simulink model "BLTSIM_MASTER_MODEL"  (R2021b)
settings: Solver=VariableStepAuto  StartTime=0.0  StopTime=Simulation.StopTime  RelTol=1e-3
undefined symbols (not defined in the file or in its folder): initialStateVector, vehicle
libraries: telemetrySubsystem x2, equationsOfMotionSubsystem x1, ForcesSubsystem x1, groundCheckSubsystem x1, outputHandlingSubsytem x1
settings Model: SnapshotInterval=1  Creator=mat  LastModifiedBy=mat

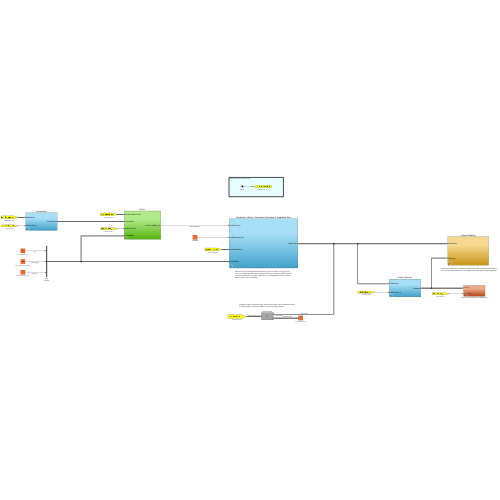
[thumbnail: Simulink's stored preview of the top-level diagram]
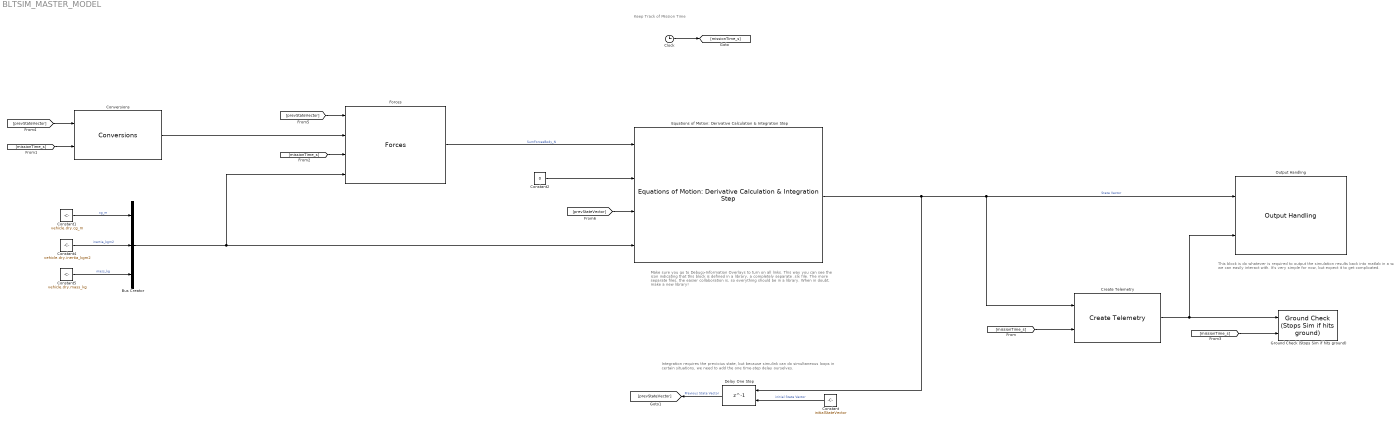
== system BLTSIM_MASTER_MODEL ==
  note: Keep Track of Mission Time
  note: Integration requires the previoius state, but because simulink can do simultaneous loops in certain situations, we need to add the one time-step delay ourselves.
  note: This block is do whatever is required to output the simulation results back into matlab in a way we can easily interact with. It's very simple for now, but expect it to get complicated.
  note: Make sure you go to Debug>Information Overlays to turn on all links. This way you can see the icon indicating that this block is defined in a library, a completely separate .slx file. The more separate files, the easier collaboration is, so everything should be in a library. When in doubt, make a new library!
  Bus Creator : BusCreator  Inputs=3  OutDataTypeStr=Bus: vehicleState_BusType  NonVirtualBus=on
      settings: InheritFromInputs=off
  Clock : Clock
  Constant : Constant  Value=initialStateVector  OutDataTypeStr=Bus: StateVector_BusType
      settings: AttributesFormatString=%<Value>
  Constant1 : Constant  Value=vehicle.dry.cg_m
      settings: AttributesFormatString=%<Value>
  Constant2 : Constant  Value=0
  Constant4 : Constant  Value=vehicle.dry.inertia_kgm2
      settings: AttributesFormatString=%<Value>
  Constant5 : Constant  Value=vehicle.dry.mass_kg
      settings: AttributesFormatString=%<Value>
  Conversions : telemetrySubsystem/Conversions  SystemSampleTime=-1  VariantActivationTime=update diagram  Latency=0  AutoFrameSizeCalculation=off
  Create Telemetry : telemetrySubsystem/Create Telemetry  SystemSampleTime=-1  VariantActivationTime=update diagram  Latency=0  AutoFrameSizeCalculation=off
  Delay One Step : Delay  DelayLength=1  InitialConditionSource=Input port
      settings: InputPortMap=u0,p4
  Equations of Motion: Derivative Calculation & Integration Step : equationsOfMotionSubsystem/Equations of Motion: Derivative Calculation & Integration Step  SystemSampleTime=-1  VariantActivationTime=update diagram  Latency=0  AutoFrameSizeCalculation=off
  Forces : ForcesSubsystem/Forces  SystemSampleTime=-1  VariantActivationTime=update diagram  Latency=0  AutoFrameSizeCalculation=off
  Ground Check (Stops Sim if hits ground) : groundCheckSubsystem/Ground Check (Stops Sim if hits ground)  SystemSampleTime=-1  VariantActivationTime=update diagram  Latency=0  AutoFrameSizeCalculation=off
  Output Handling : outputHandlingSubsytem/Output Handling  SystemSampleTime=-1  VariantActivationTime=update diagram  Latency=0  AutoFrameSizeCalculation=off
  wires:
  Equations of Motion: Derivative Calculation & Integration Step/1 -> Delay One Step/1, Create Telemetry/1, Output Handling/1  "State Vector"
  Constant/1 -> Delay One Step/2  "initial State Vector"
  Forces/1 -> Equations of Motion: Derivative Calculation & Integration Step/1  "SumForcesBody_N"
  Constant2/1 -> Equations of Motion: Derivative Calculation & Integration Step/2
  Clock/1 -> [missionTime_s]
  [missionTime_s] -> Create Telemetry/2
  Create Telemetry/1 -> Output Handling/2, Ground Check (Stops Sim if hits ground)/1
  [missionTime_s] -> Conversions/2
  Conversions/1 -> Forces/2
  [missionTime_s] -> Forces/3
  [missionTime_s] -> Ground Check (Stops Sim if hits ground)/2
  Delay One Step/1 -> [prevStateVector]  "Previous State Vector"
  [prevStateVector] -> Conversions/1
  [prevStateVector] -> Forces/1
  [prevStateVector] -> Equations of Motion: Derivative Calculation & Integration Step/3
  Constant1/1 -> Bus Creator/1  "cg_m"
  Constant4/1 -> Bus Creator/2  "inertia_kgm2"
  Constant5/1 -> Bus Creator/3  "mass_kg"
  Bus Creator/1 -> Forces/4, Equations of Motion: Derivative Calculation & Integration Step/4
